simulink model "edge1x1_toggleable"  (R2021a)
settings: Solver=VariableStepAuto  StartTime=0.0  StopTime=10.0  RelTol=1e-3
undefined symbols (not defined in the file or in its folder): Rk
libraries: simulink x1
settings Model: OrderedModelArguments=off  Creator=phill  LastModifiedBy=phill

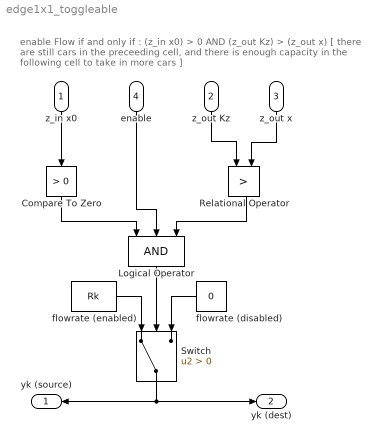
== system edge1x1_toggleable ==
  note: enable Flow if and only if : (z_in x0) > 0 AND (z_out Kz) > (z_out x)
      | [ there are still cars in the preceeding cell, and there is enough capacity
      | in the following cell to take in more cars ]
  z_in x0 : Inport
  z_out Kz : Inport  Port=2
  z_out x : Inport  Port=3
  enable : Inport  Port=4
  Compare To Zero : simulink/Logic and Bit Operations/Compare To Zero  relop=>  OutDataTypeStr=boolean
  Logical Operator : Logic  Inputs=3  AllPortsSameDT=off  OutDataTypeStr=boolean
  Relational Operator : RelationalOperator  Operator=>  OutDataTypeStr=boolean  RndMeth=Simplest
  Switch : Switch  Criteria=u2 > Threshold
  flowrate (disabled) : Constant  Value=0
  flowrate (enabled) : Constant  Value=Rk
  yk (source) : Outport
  yk (dest) : Outport  Port=2
  wires:
  Logical Operator/1 -> Switch/2
  flowrate (disabled)/1 -> Switch/3
  flowrate (enabled)/1 -> Switch/1
  Relational Operator/1 -> Logical Operator/3
  z_out x/1 -> Relational Operator/2
  Compare To Zero/1 -> Logical Operator/1
  z_in x0/1 -> Compare To Zero/1
  Switch/1 -> yk (source)/1, yk (dest)/1
  z_out Kz/1 -> Relational Operator/1
  enable/1 -> Logical Operator/2
